simulink model "sl_pursuit"  (Simulink 7.7)
settings: Solver=ode3  StartTime=0.0  StopTime=200  FixedStep=0.2  RelTol=1e-3
libraries: roblocks x3, simulink_need_slupdate x1, simulink x1
settings Model: Creator=pic  LastModifiedBy=corkep
settings DataIOCC: LimitDataPoints=off  ReturnWorkspaceOutputs=on
settings DebuggingCC: StrictBusMsg=Warning

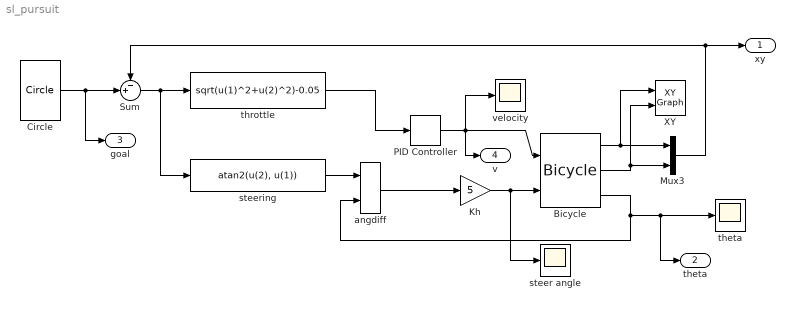
== system sl_pursuit ==
  Bicycle : roblocks/Bicycle  SystemSampleTime=-1  accel=Inf  vlim=5  alim=Inf  x0=[0, 0, 0]  handbrake=0
  Circle : roblocks/Circle  SystemSampleTime=-1  radius=1  freq=0.1
  Kh : Gain  Gain=5
  Mux3 : Mux  Inputs=2
  PID Controller : simulink_need_slupdate/PID Controller  SystemSampleTime=-1  P=1  I=0.5  D=0
  Sum : Sum  Inputs=-+|
  XY : simulink/Sinks/XY Graph  SystemSampleTime=-1  xmin=-2  xmax=2  ymin=-2  ymax=2  st=-1
  angdiff : roblocks/angdiff  SystemSampleTime=-1
  steer angle : Scope
      settings: YMin=0  YMax=4.25  SaveName=ScopeData2
  steering : Fcn  Expr=atan2(u(2), u(1))
  "theta " : Scope
  throttle : Fcn  Expr=sqrt(u(1)^2+u(2)^2)-0.05
  velocity : Scope
      settings: YMin=0.05  YMax=0.475
  xy : Outport
  theta : Outport  Port=2
  goal : Outport  Port=3
  v : Outport  Port=4
  wires:
  Bicycle/1 -> Mux3/1, XY/1
  Bicycle/2 -> Mux3/2, XY/2
  Circle/1 -> Sum/2, goal/1
  Mux3/1 -> Sum/1, xy/1
  Sum/1 -> throttle/1, steering/1
  throttle/1 -> PID Controller/1
  steering/1 -> angdiff/1
  Bicycle/3 -> "theta "/1, theta/1, angdiff/2
  angdiff/1 -> Kh/1
  Kh/1 -> Bicycle/2, steer angle/1
  PID Controller/1 -> velocity/1, Bicycle/1, v/1
